simulink model "TVModel"  (R2022a)
settings: Solver=FixedStepDiscrete  StartTime=0.0  StopTime=10.0  FixedStep=0.02  MaxStep=0.01  RelTol=1e-3
undefined symbols (not defined in the file or in its folder): MB, TV, TV_OLD
libraries: simulink x22, simulink_extras x14, slpidlib x8, fuzblock x5, controlLib x4, dspstat3 x4, eeGeneralControl x3, cstblocks x3, eeSlidingModeController x1, sharedTrackingLibrary x1
(part 4 of 8)

== system TVModel/Subsystem/Subsystem1/Torque Distribution/Reference Tracking/YRD_LUT_-3 ==
  front_wheel_angle : Inport
  vx : Inport  Port=2
  Action Port : ActionPort  ActionPortLabel=elseif(u1 ==4)
  Abs : Abs  SaturateOnIntegerOverflow=off
  Cast3 : DataTypeConversion  Commented=on  OutDataTypeStr=single  SaturateOnIntegerOverflow=off  RndMeth=Floor
  Divide : Product  Inputs=*/
  Divide1 : Product  Inputs=*/
  Divide2 : Product  Inputs=**
  LUT_-3 : Lookup_n-D  BreakpointsForDimension1=TV.LUT.Yrd_LUT.LUT_vectors.delta_vector  BreakpointsForDimension2=TV.LUT.Yrd_LUT.LUT_vectors.v_vector  Table=single(TV.LUT.Yrd_LUT.LUT_neg3.ay_matrix)  InternalRulePriority=Speed  RndMeth=Simplest
      settings: InputPortMap=u0,u1
  Saturation : Saturate  UpperLimit=inf  LowerLimit=3
  yrd : Outport
  wires:
  front_wheel_angle/1 -> Divide1/1, Abs/1
  Abs/1 -> Divide1/2, LUT_-3/1  "absolute_front_wheel_angle"
  Divide/1 -> Divide2/2
  LUT_-3/1 -> Divide/1  "a"
  vx/1 -> Saturation/1
  Saturation/1 -> Divide/2, LUT_-3/2  "vx"
  Divide2/1 -> yrd/1  "yrd"
  Divide1/1 -> Divide2/1  "normalized_front_wheel_angle"

== system TVModel/Subsystem/Subsystem1/Torque Distribution/Reference Tracking/YRD_LUT_0 ==
  front_wheel_angle : Inport
  vx : Inport  Port=2
  Action Port : ActionPort  ActionPortLabel=elseif(u1 ==2)
  Abs : Abs  SaturateOnIntegerOverflow=off
  Cast : DataTypeConversion  Commented=on  OutDataTypeStr=single  SaturateOnIntegerOverflow=off  RndMeth=Floor
  Divide : Product  Inputs=*/
  Divide1 : Product  Inputs=*/
  Divide2 : Product  Inputs=**
  LUT_0 : Lookup_n-D  BreakpointsForDimension1=TV.LUT.Yrd_LUT.LUT_vectors.delta_vector  BreakpointsForDimension2=TV.LUT.Yrd_LUT.LUT_vectors.v_vector  Table=single(TV.LUT.Yrd_LUT.LUT_0.ay_matrix)  InternalRulePriority=Speed  RndMeth=Simplest
      settings: InputPortMap=u0,u1
  Saturation : Saturate  UpperLimit=inf  LowerLimit=3
  yrd : Outport
  wires:
  front_wheel_angle/1 -> Divide1/1, Abs/1
  Saturation/1 -> Divide/2, LUT_0/2  "vx"
  Abs/1 -> Divide1/2, LUT_0/1  "absolute_front_wheel_angle"
  Divide2/1 -> yrd/1  "yrd"
  vx/1 -> Saturation/1
  Divide/1 -> Divide2/2
  Divide1/1 -> Divide2/1  "normalized_front_wheel_angle"
  LUT_0/1 -> Divide/1

== system TVModel/Subsystem/Subsystem1/Torque Distribution/Reference Tracking/YRD_LUT_1 ==
  front_wheel_angle : Inport
  vx : Inport  Port=2
  Action Port : ActionPort  ActionPortLabel=if(u1 == 1)
  Abs : Abs  SaturateOnIntegerOverflow=off
  Cast3 : DataTypeConversion  Commented=on  OutDataTypeStr=single  SaturateOnIntegerOverflow=off  RndMeth=Floor
  Divide : Product  Inputs=*/
  Divide1 : Product  Inputs=*/
  Divide2 : Product  Inputs=**
  LUT_1 : Lookup_n-D  BreakpointsForDimension1=TV.LUT.Yrd_LUT.LUT_vectors.delta_vector  BreakpointsForDimension2=TV.LUT.Yrd_LUT.LUT_vectors.v_vector  Table=single(TV.LUT.Yrd_LUT.LUT_1.ay_matrix)  InternalRulePriority=Speed  RndMeth=Simplest
      settings: InputPortMap=u0,u1
  Saturation : Saturate  UpperLimit=inf  LowerLimit=3
  yrd : Outport
  wires:
  front_wheel_angle/1 -> Divide1/1, Abs/1
  LUT_1/1 -> Divide/1
  vx/1 -> Saturation/1
  Divide1/1 -> Divide2/1  "normalized_front_wheel_angle"
  Divide2/1 -> yrd/1  "yrd"
  Abs/1 -> Divide1/2, LUT_1/1  "absolute_front_wheel_angle"
  Saturation/1 -> Divide/2, LUT_1/2  "vx"
  Divide/1 -> Divide2/2

== system TVModel/Subsystem/Subsystem1/Torque Distribution/Reference Tracking/YRD_LUT_2 ==
  front_wheel_angle : Inport
  vx : Inport  Port=2
  Action Port : ActionPort  ActionPortLabel=elseif(u1 ==2)
  Abs : Abs  SaturateOnIntegerOverflow=off
  Cast : DataTypeConversion  Commented=on  OutDataTypeStr=single  SaturateOnIntegerOverflow=off  RndMeth=Floor
  Divide : Product  Inputs=*/
  Divide1 : Product  Inputs=*/
  Divide2 : Product  Inputs=**
  LUT_0 : Lookup_n-D  BreakpointsForDimension1=TV.LUT.Yrd_LUT.LUT_vectors.delta_vector  BreakpointsForDimension2=TV.LUT.Yrd_LUT.LUT_vectors.v_vector  Table=single(TV.LUT.Yrd_LUT.LUT_0.ay_matrix)  InternalRulePriority=Speed  RndMeth=Simplest
      settings: InputPortMap=u0,u1
  Saturation : Saturate  UpperLimit=inf  LowerLimit=3
  yrd : Outport
  wires:
  LUT_0/1 -> Divide/1
  Divide1/1 -> Divide2/1  "normalized_front_wheel_angle"
  Divide/1 -> Divide2/2
  vx/1 -> Saturation/1
  Divide2/1 -> yrd/1  "yrd"
  Abs/1 -> LUT_0/1, Divide1/2  "absolute_front_wheel_angle"
  Saturation/1 -> LUT_0/2, Divide/2  "vx"
  front_wheel_angle/1 -> Abs/1, Divide1/1

== system TVModel/Subsystem/Subsystem1/Torque Distribution/Reference Tracking/YRD_LUT_3 ==
  front_wheel_angle : Inport
  vx : Inport  Port=2
  Action Port : ActionPort  ActionPortLabel=if(u1 == 1)
  Abs : Abs  SaturateOnIntegerOverflow=off
  Cast3 : DataTypeConversion  Commented=on  OutDataTypeStr=single  SaturateOnIntegerOverflow=off  RndMeth=Floor
  Divide : Product  Inputs=*/
  Divide1 : Product  Inputs=*/
  Divide2 : Product  Inputs=**
  LUT_1 : Lookup_n-D  BreakpointsForDimension1=TV.LUT.Yrd_LUT.LUT_vectors.delta_vector  BreakpointsForDimension2=TV.LUT.Yrd_LUT.LUT_vectors.v_vector  Table=single(TV.LUT.Yrd_LUT.LUT_1.ay_matrix)  InternalRulePriority=Speed  RndMeth=Simplest
      settings: InputPortMap=u0,u1
  Saturation : Saturate  UpperLimit=inf  LowerLimit=3
  yrd : Outport
  wires:
  Divide/1 -> Divide2/2
  Saturation/1 -> LUT_1/2, Divide/2  "vx"
  Abs/1 -> LUT_1/1, Divide1/2  "absolute_front_wheel_angle"
  Divide2/1 -> yrd/1  "yrd"
  Divide1/1 -> Divide2/1  "normalized_front_wheel_angle"
  vx/1 -> Saturation/1
  LUT_1/1 -> Divide/1
  front_wheel_angle/1 -> Abs/1, Divide1/1

== system TVModel/Subsystem/Subsystem1/Torque Limits/Torque Limits Positive/Torque_Curve ==
  omega_wheels : Inport
  voltage [ID380] : Inport  Port=2
  torque_map : Inport  Port=3
  2-D Lookup Table : Lookup_n-D  BreakpointsForDimension1=TV.LV.TORQUE.T_lim_pos.breakpoints1  BreakpointsForDimension2=TV.LV.TORQUE.T_lim_pos.breakpoints2  Table=TV.LV.TORQUE.T_lim_pos.table_data  ExtrapMethod=Clip  InternalRulePriority=Speed  OutDataTypeStr=double  RndMeth=Simplest
      settings: InputPortMap=u0,u1
  Constant : Constant  Value=0
  Constant1 : Constant  Value=TV.LV.TORQUE.T_peak_motor
  Constant2 : Constant  Value=TV.LV.TORQUE.T_nominal_motor
  Gain : Gain  Gain=TV.LV.TORQUE.T_nominal_motor/1000
  Gain4 : Gain  Gain=TV.CAR.Tau*60/(2*pi)
  Low-Pass Filter (Discrete or Continuous) : eeGeneralControl/Low-Pass Filter (Discrete or Continuous)  K=1  T=1/4/pi  B=inf  A=-inf  init_option=Inherited from block input  x0=0  Ts=TV.MPC.T/TV.MPC.N
  Multiport Switch : MultiPortSwitch  DataPortOrder=Specify indices  DataPortIndices={TV.LV.TORQUE.T_peak_setting,TV.LV.TORQUE.T_nominal_setting}  DiagnosticForDefault=None  SaturateOnIntegerOverflow=off  InputSameDT=off
  Saturation Dynamic : simulink/Discontinuities/Saturation Dynamic  OutMin=[]  OutMax=[]  OutDataTypeStr=Inherit: Same as second input  OutDataType=fixdt(1, 16)  OutScaling=2^-10  DoSatur=off
  Saturation1 : Saturate  UpperLimit=+inf  LowerLimit=0
  max_torque_available : Outport
  wires:
  Low-Pass Filter (Discrete or Continuous)/1 -> Saturation Dynamic/2
  omega_wheels/1 -> Gain4/1
  Constant/1 -> Saturation Dynamic/3
  torque_map/1 -> Multiport Switch/1
  Constant1/1 -> Multiport Switch/2
  Constant2/1 -> Multiport Switch/3
  Multiport Switch/1 -> Saturation Dynamic/1  "torque map selected"
  Saturation1/1 -> 2-D Lookup Table/1
  voltage [ID380]/1 -> 2-D Lookup Table/2
  Gain/1 -> Low-Pass Filter (Discrete or Continuous)/1
  2-D Lookup Table/1 -> Gain/1
  Gain4/1 -> Saturation1/1  "RPM_Motors"
  Saturation Dynamic/1 -> max_torque_available/1

== system TVModel/Subsystem/Subsystem1/Torque Limits/Torque Limits Regen/Torque_Curve ==
  omega_wheels : Inport
  voltage [ID380] : Inport  Port=2
  torque_map : Inport  Port=3
  2-D Lookup Table : Lookup_n-D  BreakpointsForDimension1=TV.LV.TORQUE.T_lim_pos.breakpoints1  BreakpointsForDimension2=TV.LV.TORQUE.T_lim_pos.breakpoints2  Table=TV.LV.TORQUE.T_lim_pos.table_data  ExtrapMethod=Clip  InternalRulePriority=Speed  OutDataTypeStr=double  RndMeth=Simplest
      settings: InputPortMap=u0,u1
  Constant : Constant  Value=0
  Constant1 : Constant  Value=TV.LV.TORQUE.T_peak_motor
  Constant2 : Constant  Value=TV.LV.TORQUE.T_nominal_motor
  Gain : Gain  Gain=TV.LV.TORQUE.T_nominal_motor/1000
  Gain4 : Gain  Gain=TV.CAR.Tau*60/(2*pi)
  Low-Pass Filter (Discrete or Continuous) : eeGeneralControl/Low-Pass Filter (Discrete or Continuous)  K=1  T=1/4/pi  B=inf  A=-inf  init_option=Inherited from block input  x0=0  Ts=TV.MPC.T/TV.MPC.N
  Multiport Switch : MultiPortSwitch  DataPortOrder=Specify indices  DataPortIndices={TV.LV.TORQUE.T_peak_setting,TV.LV.TORQUE.T_nominal_setting}  DiagnosticForDefault=None  SaturateOnIntegerOverflow=off  InputSameDT=off
  Saturation Dynamic : simulink/Discontinuities/Saturation Dynamic  OutMin=[]  OutMax=[]  OutDataTypeStr=Inherit: Same as second input  OutDataType=fixdt(1, 16)  OutScaling=2^-10  DoSatur=off
  Saturation1 : Saturate  UpperLimit=+inf  LowerLimit=0
  max_torque_available : Outport
  wires:
  Low-Pass Filter (Discrete or Continuous)/1 -> Saturation Dynamic/2
  omega_wheels/1 -> Gain4/1
  Constant/1 -> Saturation Dynamic/3
  torque_map/1 -> Multiport Switch/1
  Constant1/1 -> Multiport Switch/2
  Constant2/1 -> Multiport Switch/3
  Multiport Switch/1 -> Saturation Dynamic/1  "torque map selected"
  Saturation1/1 -> 2-D Lookup Table/1
  voltage [ID380]/1 -> 2-D Lookup Table/2
  Gain/1 -> Low-Pass Filter (Discrete or Continuous)/1
  2-D Lookup Table/1 -> Gain/1
  Gain4/1 -> Saturation1/1  "RPM_Motors"
  Saturation Dynamic/1 -> max_torque_available/1

== system TVModel/Subsystem/Subsystem1/Torque Limits/Torque Request/T_Req_Acceleration ==
  throttle : Inport
  torque_map : Inport  Port=2
  Constant : Constant  Value=0
  Constant1 : Constant
  Constant2 : Constant  Value=0
  Data Store General_Params : DataStoreRead  DataStoreName=General_Params  DataStoreElements=General_Params.ThrottleThresh  IndexOptions=Index vector (dialog)  Indices=1  OutputSizes=1
  Data Store General_Params1 : DataStoreRead  DataStoreName=General_Params  DataStoreElements=General_Params.ThrottleThresh  IndexOptions=Index vector (dialog)  Indices=1  OutputSizes=1
  Less Than : RelationalOperator  Operator=>  OutDataTypeStr=boolean  RndMeth=Simplest  InputSameDT=off
  Map_Selector : MultiPortSwitch  DataPortOrder=Specify indices  DataPortIndices={TV.LV.TORQUE.T_peak_setting,TV.LV.TORQUE.T_nominal_setting}  DiagnosticForDefault=None  SaturateOnIntegerOverflow=off  InputSameDT=off
  Mux : Mux  Inputs=3
  Switch : Switch  Criteria=u2 > Threshold  SaturateOnIntegerOverflow=off  InputSameDT=off
  T_nominal_wheel_LUT : Lookup_n-D  NumberOfTableDimensions=1  BreakpointsForDimension1Source=Input port  BreakpointsForDimension1=[-5:5]  Table=[0,0, 4*TV.LV.TORQUE.T_nominal_wheel]  InternalRulePriority=Speed  RndMeth=Simplest
      settings: InputPortMap=u0,p5
  T_peak_wheel_LUT : Lookup_n-D  NumberOfTableDimensions=1  BreakpointsForDimension1Source=Input port  BreakpointsForDimension1=[-5:5]  Table=[0,0, 4*TV.LV.TORQUE.T_peak_wheel]  InternalRulePriority=Speed  RndMeth=Simplest
      settings: InputPortMap=u0,p5
  "t_req " : Outport
  wires:
  throttle/1 -> T_nominal_wheel_LUT/1, Less Than/1, T_peak_wheel_LUT/1  "throttle"
  Map_Selector/1 -> Switch/1  "t"
  Data Store General_Params1/1 -> Less Than/2  "throttle_thresh"
  Less Than/1 -> Switch/2  "throttle"
  Switch/1 -> "t_req "/1
  Constant/1 -> Switch/3
  T_nominal_wheel_LUT/1 -> Map_Selector/3
  T_peak_wheel_LUT/1 -> Map_Selector/2
  torque_map/1 -> Map_Selector/1  "torque_map"
  Mux/1 -> T_nominal_wheel_LUT/2, T_peak_wheel_LUT/2
  Data Store General_Params/1 -> Mux/2  "throttle_thresh"
  Constant1/1 -> Mux/3
  Constant2/1 -> Mux/1

== system TVModel/Subsystem/Subsystem1/Torque Limits/Torque Request/T_Req_Braking ==
  brake : Inport
  1-D Lookup Table : Lookup_n-D  NumberOfTableDimensions=1  BreakpointsForDimension1Source=Input port  BreakpointsForDimension1=[-5:5]  Table=[0,1]  InternalRulePriority=Speed  RndMeth=Simplest
      settings: InputPortMap=u0,p5
  Constant : Constant
  Data Store Read : DataStoreRead  DataStoreName=General_Params  DataStoreElements=General_Params.BrakeThresh  IndexOptions=Index vector (dialog)  Indices=1  OutputSizes=1
  Gain_Max_Torque_Needed : Gain  Gain=-4*TV.LV.TORQUE.T_nominal_wheel
  Mux : Mux  Inputs=2
  Saturation_Brake : Saturate  UpperLimit=1  LowerLimit=0
  "t_req " : Outport
  wires:
  Gain_Max_Torque_Needed/1 -> "t_req "/1  "t_req"
  brake/1 -> 1-D Lookup Table/1  "brake"
  1-D Lookup Table/1 -> Saturation_Brake/1  "brake"
  Saturation_Brake/1 -> Gain_Max_Torque_Needed/1  "brake"
  Data Store Read/1 -> Mux/1
  Constant/1 -> Mux/2
  Mux/1 -> 1-D Lookup Table/2

== system TVModel/Subsystem/Subsystem1/Slip Control/Traction Control/Load Transfer calculation/Fz FL ==
  In Bus Element : Inport  PortName=dynamics_data  Element=ay
  In Bus Element1 : Inport  PortName=dynamics_data  Element=vx
  In Bus Element2 : Inport  PortName=dynamics_data  Element=ax
  Drag moment : Gain  Gain=0.5*TV.CAR.rho*TV.CAR.CdA*TV.CAR.hcop/TV.CAR.wb*0.5
  Lateral Load Transfer : Gain  Gain=TV.CAR.m/TV.CAR.tf*TV.CAR.hcog*0.5*0.5
  Lift Force : Gain  Gain=0.5*TV.CAR.rho*TV.CAR.ClA*(1-TV.CAR.xcop/TV.CAR.wb)*0.5
  Longitudinal Load Transfer : Gain  Gain=TV.CAR.m/TV.CAR.wb*TV.CAR.hcog*0.5
  Square1 : Math  Operator=square
  Square2 : Math  Operator=square
  Static Load Front : Constant  Value=TV.CAR.Fzf
  Subtract : Sum  Inputs=+++-+
  Unary Minus : UnaryMinus
  Unary Minus1 : UnaryMinus
  TV_Info : Outport
  wires:
  Unary Minus1/1 -> Longitudinal Load Transfer/1
  Unary Minus/1 -> Lateral Load Transfer/1
  In Bus Element/1 -> Unary Minus/1
  Subtract/1 -> TV_Info/1
  Drag moment/1 -> Subtract/4
  Static Load Front/1 -> Subtract/1
  Square1/1 -> Lift Force/1
  Lateral Load Transfer/1 -> Subtract/2
  Longitudinal Load Transfer/1 -> Subtract/5
  In Bus Element2/1 -> Unary Minus1/1
  Square2/1 -> Drag moment/1
  In Bus Element1/1 -> Square2/1, Square1/1
  Lift Force/1 -> Subtract/3

== system TVModel/Subsystem/Subsystem1/Slip Control/Traction Control/Load Transfer calculation/Fz FR ==
  In Bus Element : Inport  PortName=dynamics_data  Element=ay
  In Bus Element1 : Inport  PortName=dynamics_data  Element=vx
  In Bus Element2 : Inport  PortName=dynamics_data  Element=ax
  Drag moment : Gain  Gain=0.5*TV.CAR.rho*TV.CAR.CdA*TV.CAR.hcop/TV.CAR.wb*0.5
  Lateral Load Transfer : Gain  Gain=TV.CAR.m/TV.CAR.tf*TV.CAR.hcog*0.5*0.5
  Lift Force : Gain  Gain=0.5*TV.CAR.rho*TV.CAR.ClA*(1 - TV.CAR.xcop/TV.CAR.wb)*0.5
  Longitudinal Load Transfer : Gain  Gain=TV.CAR.m/TV.CAR.wb*TV.CAR.hcog*0.5
  Square1 : Math  Operator=square
  Square2 : Math  Operator=square
  Static Load Front : Constant  Value=TV.CAR.Fzf
  Subtract : Sum  Inputs=+-+-+
  Unary Minus : UnaryMinus
  Unary Minus1 : UnaryMinus
  TV_Info : Outport
  wires:
  Unary Minus1/1 -> Longitudinal Load Transfer/1
  Unary Minus/1 -> Lateral Load Transfer/1
  Subtract/1 -> TV_Info/1
  Drag moment/1 -> Subtract/4
  In Bus Element/1 -> Unary Minus/1
  In Bus Element1/1 -> Square1/1, Square2/1
  Static Load Front/1 -> Subtract/1
  Square1/1 -> Lift Force/1
  Lateral Load Transfer/1 -> Subtract/2
  Longitudinal Load Transfer/1 -> Subtract/5
  In Bus Element2/1 -> Unary Minus1/1
  Lift Force/1 -> Subtract/3
  Square2/1 -> Drag moment/1

== system TVModel/Subsystem/Subsystem1/Slip Control/Traction Control/Load Transfer calculation/Fz RL ==
  In Bus Element : Inport  PortName=dynamics_data  Element=ay
  In Bus Element1 : Inport  PortName=dynamics_data  Element=vx
  In Bus Element2 : Inport  PortName=dynamics_data  Element=ax
  Drag moment : Gain  Gain=0.5*TV.CAR.rho*TV.CAR.CdA*TV.CAR.hcop/TV.CAR.wb*0.5
  Lateral Load Transfer : Gain  Gain=TV.CAR.m/TV.CAR.tr*TV.CAR.hcog*0.5*0.5
  Lift Force : Gain  Gain=0.5*TV.CAR.rho*TV.CAR.ClA*(TV.CAR.xcop/TV.CAR.wb)*0.5
  Longitudinal Load Transfer : Gain  Gain=TV.CAR.m/TV.CAR.wb*TV.CAR.hcog*0.5
  Square1 : Math  Operator=square
  Square2 : Math  Operator=square
  Static Load Front : Constant  Value=TV.CAR.Fzr
  Subtract : Sum  Inputs=++++-
  Unary Minus : UnaryMinus
  Unary Minus1 : UnaryMinus
  TV_Info : Outport
  wires:
  Unary Minus1/1 -> Longitudinal Load Transfer/1
  Unary Minus/1 -> Lateral Load Transfer/1
  Subtract/1 -> TV_Info/1
  Drag moment/1 -> Subtract/4
  In Bus Element/1 -> Unary Minus/1
  Static Load Front/1 -> Subtract/1
  Square1/1 -> Lift Force/1
  Lateral Load Transfer/1 -> Subtract/2
  Longitudinal Load Transfer/1 -> Subtract/5
  In Bus Element2/1 -> Unary Minus1/1
  Lift Force/1 -> Subtract/3
  Square2/1 -> Drag moment/1
  In Bus Element1/1 -> Square2/1, Square1/1

== system TVModel/Subsystem/Subsystem1/Slip Control/Traction Control/Load Transfer calculation/Fz RR ==
  In Bus Element : Inport  PortName=dynamics_data  Element=ay
  In Bus Element1 : Inport  PortName=dynamics_data  Element=vx
  In Bus Element2 : Inport  PortName=dynamics_data  Element=ax
  Drag moment : Gain  Gain=0.5*TV.CAR.rho*TV.CAR.CdA*TV.CAR.hcop/TV.CAR.wb*0.5
  Lateral Load Transfer : Gain  Gain=TV.CAR.m/TV.CAR.tr*TV.CAR.hcog*0.5*0.5
  Lift Force : Gain  Gain=0.5*TV.CAR.rho*TV.CAR.ClA*(TV.CAR.xcop/TV.CAR.wb)*0.5
  Longitudinal Load Transfer : Gain  Gain=TV.CAR.m/TV.CAR.wb*TV.CAR.hcog*0.5
  Square1 : Math  Operator=square
  Square2 : Math  Operator=square
  Static Load Front : Constant  Value=TV.CAR.Fzr
  Subtract : Sum  Inputs=+-++-
  Unary Minus : UnaryMinus
  Unary Minus1 : UnaryMinus
  TV_Info : Outport
  wires:
  Unary Minus1/1 -> Longitudinal Load Transfer/1
  Unary Minus/1 -> Lateral Load Transfer/1
  Subtract/1 -> TV_Info/1
  Drag moment/1 -> Subtract/4
  In Bus Element/1 -> Unary Minus/1
  In Bus Element1/1 -> Square1/1, Square2/1
  Static Load Front/1 -> Subtract/1
  Square1/1 -> Lift Force/1
  Lateral Load Transfer/1 -> Subtract/2
  Longitudinal Load Transfer/1 -> Subtract/5
  In Bus Element2/1 -> Unary Minus1/1
  Lift Force/1 -> Subtract/3
  Square2/1 -> Drag moment/1

== system TVModel/Subsystem/Subsystem1/Slip Control/Traction Control/S-R Flip Flops/Subsystem ==
  In1 : Inport
  In2 : Inport  Port=2
  Demux : Demux
  Demux1 : Demux
  Mux : Mux
  S-R Flip-Flop{,1..3} (4 alike) : simulink_extras/Flip Flops/S-R Flip-Flop  initial_condition=0
  Out1 : Outport
  wires:
  Demux1/1 -> S-R Flip-Flop/2
  Demux1/2 -> S-R Flip-Flop1/2
  Demux/4 -> S-R Flip-Flop3/1
  Demux/1 -> S-R Flip-Flop/1
  In1/1 -> Demux/1
  Demux1/3 -> S-R Flip-Flop2/2
  Demux/2 -> S-R Flip-Flop1/1
  Demux1/4 -> S-R Flip-Flop3/2
  S-R Flip-Flop2/1 -> Mux/3
  Demux/3 -> S-R Flip-Flop2/1
  S-R Flip-Flop3/1 -> Mux/4
  In2/1 -> Demux1/1
  Mux/1 -> Out1/1
  S-R Flip-Flop1/1 -> Mux/2
  S-R Flip-Flop/1 -> Mux/1

== system TVModel/Subsystem/Subsystem1/Slip Control/Traction Control/Slip Control/ABS ==
  eps_target : Inport
  eps : Inport  Port=2
  Reset Signal : Inport  Port=3
  T_actual : Inport  Port=4  PortDimensions=4
  T_limit : Inport  Port=5
  RTD_flag : Inport  Port=6
  Activation logic : Stateflow chart  TreatAsAtomicUnit=on
  Constant : Constant  Value=0.01
  Constant1 : Constant  Value=57
  Constant2 : Constant  Value=2845
  Constant3 : Constant  Value=4.9
  Constant4 : Constant  Value=-21
  Constant5 : Constant  Value=0.9
  Gain : Gain  Gain=-1
  Minus : Sum  Inputs=+-
  PID Controller5 : slpidlib/PID Controller  Controller=PI  Form=Parallel  TimeDomain=Discrete-time  UseExternalTs=off  SampleTime=0.02  IntegratorMethod=Forward Euler  FilterMethod=Forward Euler  ControllerParametersSource=external  P=57  I=2845  UseKiTs=off  D=0  N=63.8249907657072  UseFilter=off  TunerSelectOption=Transfer Function Based (PID Tuner App)  InitialConditionSource=internal  InitialConditionForIntegrator=0  InitialConditionForFilter=0  DifferentiatorICPrevScaledInput=0  ExternalReset=rising  TrackingMode=on  Kt=TV_OLD.LV.GEN.slipKt  LimitOutput=on  SatLimitsSource=external  UpperSaturationLimit=0  LowerSaturationLimit=-TV_OLD.LV.Tpeak  LinearizeAsGain=on  AntiWindupMode=clamping  Kb=1  POutMin=[]  POutMax=[]  IOutMin=[]  IOutMax=[]  DOutMin=[]  DOutMax=[]  NOutMin=[]  NOutMax=[]  SumOutMin=[]  SumOutMax=[]  SaturationOutMin=[]  SaturationOutMax=[]  PParamMin=[]  PParamMax=[]  IParamMin=[]  IParamMax=[]  DParamMin=[]  DParamMax=[]  NParamMin=[]  NParamMax=[]  KbParamMin=[]  KbParamMax=[]  KtParamMin=[]  KtParamMax=[]  KbOutMin=[]  KbOutMax=[]  KtOutMin=[]  KtOutMax=[]  IntegratorOutMin=[]  IntegratorOutMax=[]  FilterOutMin=[]  FilterOutMax=[]  SumI1OutMin=[]  SumI1OutMax=[]  SumI2OutMin=[]  SumI2OutMax=[]  SumI3OutMin=[]  SumI3OutMax=[]  SumI4OutMin=[]  SumI4OutMax=[]  SumDOutMin=[]  SumDOutMax=[]  DifferentiatorOutMin=[]  DifferentiatorOutMax=[]  FilterDiffOutCoefMin=[]  FilterDiffOutCoefMax=[]  ReciprocalOutMin=[]  ReciprocalOutMax=[]  SumDenOutMin=[]  SumDenOutMax=[]  SumNumOutMin=[]  SumNumOutMax=[]  DivideOutMin=[]  DivideOutMax=[]  UdiffTsProdOutMin=[]  UdiffTsProdOutMax=[]  NTsProdOutMin=[]  NTsProdOutMax=[]  UintegralTsProdOutMin=[]  UintegralTsProdOutMax=[]  UngainTsProdOutMin=[]  UngainTsProdOutMax=[]  IntegratorContinuousStateAttributes=''  IntegratorStateMustResolveToSignalObject=off  IntegratorRTWStateStorageClass=Auto  FilterContinuousStateAttributes=''  FilterStateMustResolveToSignalObject=off  FilterRTWStateStorageClass=Auto  ParallelPVariant=ExternalParameters  IdealPVariant=Disabled  IVariant=ExternalParameters  DVariant=Disabled  IntegratorVariant=Discrete  SatVariant=External  AWVariant=DiscClampingParallel  PCopyVariant=Disabled  TRVariant=Enabled  FdbkBlocksVariant=Forward  IdealPFdbkVariant=Disabled  SatFdbkVariant=Disabled  DerivativeFilterVariant=Disabled  NVariant=Disabled  NCopyVariant=Disabled_SignalSpec  FilterICVariant=Disabled  IntegratorICVariant=InternalICs  ExternalResetVariant=ExternalReset  TRSumVariant=TrackingMode  SumFdbkVariant=Disabled  SumVariant=Sum_PI  TsampFilterVariant=InternalTs  TsampNgainVariant=Passthrough  TsampIntegralVariant=Passthrough  ExternalSaturationOutDataTypeStr=Inherit: Same as second input  aMode=0
  Unit Delay : UnitDelay  InitialCondition=zeros(4,1)  SampleTime=-1  HasFrameUpgradeWarning=on
  Tmin : Outport
  wires:
  Constant2/1 -> PID Controller5/3
  Constant1/1 -> PID Controller5/2
  [ResetSignal] -> Activation logic/6(TC_flag)
  [ResetSignal] -> PID Controller5/4
  Reset Signal/1 -> [ResetSignal]
  [eps] -> Activation logic/3(eps)
  [eps] -> Minus/2
  eps/1 -> [eps]
  [eps_target] -> Activation logic/2(epsTarget)
  eps_target/1 -> [eps_target]
  Minus/1 -> PID Controller5/1
  Activation logic/1(T_min) -> Tmin/1, Unit Delay/1, PID Controller5/7
  T_actual/1 -> Activation logic/4(T_actual)
  Unit Delay/1 -> Activation logic/7(Tmin_old)
  [eps_target] -> Minus/1
  PID Controller5/1 -> Activation logic/1(Tmin_PI)  "Tmin_PI"
  T_limit/1 -> Activation logic/5(T_limit)
  Constant/1 -> Activation logic/8(slipNoise)
  Constant3/1 -> Gain/1
  Gain/1 -> PID Controller5/5
  Constant4/1 -> PID Controller5/6
  Constant5/1 -> Activation logic/9(slipDeactPerc)
  RTD_flag/1 -> Activation logic/10(RTD_flag)

== system TVModel/Subsystem/Subsystem1/Slip Control/Traction Control/Slip Control/Reset ABS ==
  V : Inport
  throttle : Inport  Port=2
  brake : Inport  Port=3
  TC_setting : Inport  Port=4
  RTD : Inport  Port=5
  AND : Logic  Inputs=3  IconShape=distinctive  AllPortsSameDT=off  OutDataTypeStr=boolean
  Constant : Constant  Value=0
  Constant1 : Constant  Value=0
  Constant2 : Constant  Value=3
  Data Store Read1 : DataStoreRead  Commented=on  DataStoreName=thresholds  DataStoreElements=thresholds.THROTTLE_RELAY_AMP#thresholds.THROTTLE_NOISE#thresholds.BRAKE_RELAY_AMP#thresholds.BRAKE_NOISE  IndexOptions=Index vector (dialog)  Indices=1  OutputSizes=1
  NOT : Logic  Commented=on  Operator=NOT  IconShape=distinctive  AllPortsSameDT=off  OutDataTypeStr=boolean
  Relational Operator : RelationalOperator  Operator=>  OutDataTypeStr=boolean  RndMeth=Simplest  InputSameDT=off
  Relational Operator3 : RelationalOperator  Operator=>  OutDataTypeStr=boolean  RndMeth=Simplest  InputSameDT=off
  Relational Operator4 : RelationalOperator  Operator=>  OutDataTypeStr=boolean  RndMeth=Simplest  InputSameDT=off
  Variable Amplitude Relay : controlLib/Variable Amplitude Relay  Commented=on  SystemSampleTime=-1  VariantActivationTime=update diagram  Latency=0  AutoFrameSizeCalculation=off
      settings: SourceProductName=VCU Library
  Variable Amplitude Relay1 : controlLib/Variable Amplitude Relay  Commented=on  SystemSampleTime=-1  VariantActivationTime=update diagram  Latency=0  AutoFrameSizeCalculation=off
      settings: SourceProductName=VCU Library
  resetSignal : Outport
  wires:
  Variable Amplitude Relay/1 -> NOT/1
  brake/1 -> Variable Amplitude Relay/3
  throttle/1 -> Variable Amplitude Relay1/3
  Data Store Read1/2 -> Variable Amplitude Relay1/2
  Data Store Read1/3 -> Variable Amplitude Relay/1
  Data Store Read1/4 -> Variable Amplitude Relay/2
  AND/1 -> resetSignal/1
  Relational Operator4/1 -> AND/3
  Relational Operator3/1 -> AND/2
  Relational Operator/1 -> AND/1
  RTD/1 -> Relational Operator4/1
  Constant1/1 -> Relational Operator4/2
  Constant/1 -> Relational Operator3/2
  TC_setting/1 -> Relational Operator3/1
  Data Store Read1/1 -> Variable Amplitude Relay1/1
  V/1 -> Relational Operator/1
  Constant2/1 -> Relational Operator/2

== system TVModel/Subsystem/Subsystem1/Slip Control/Traction Control/Slip Control/Reset TC ==
  V : Inport
  throttle : Inport  Port=2
  brake : Inport  Port=3
  TC_setting : Inport  Port=4
  RTD : Inport  Port=5
  AND : Logic  Inputs=5  IconShape=distinctive  AllPortsSameDT=off  OutDataTypeStr=boolean
  Constant : Constant  Value=0
  Constant1 : Constant  Value=0
  Constant2 : Constant  Value=3
  Constant3 : Constant  Value=0.01
  Constant4 : Constant  Value=0.05
  Constant5 : Constant  Value=0.01
  Constant6 : Constant  Value=0.1
  NOT : Logic  Operator=NOT  IconShape=distinctive  AllPortsSameDT=off  OutDataTypeStr=boolean
  Relational Operator : RelationalOperator  Operator=>  OutDataTypeStr=boolean  RndMeth=Simplest  InputSameDT=off
  Relational Operator3 : RelationalOperator  Operator=>  OutDataTypeStr=boolean  RndMeth=Simplest  InputSameDT=off
  Relational Operator4 : RelationalOperator  Operator=>  OutDataTypeStr=boolean  RndMeth=Simplest  InputSameDT=off
  Variable Amplitude Relay : controlLib/Variable Amplitude Relay  SystemSampleTime=-1  VariantActivationTime=update diagram  Latency=0  AutoFrameSizeCalculation=off
      settings: SourceProductName=VCU Library
  Variable Amplitude Relay1 : controlLib/Variable Amplitude Relay  SystemSampleTime=-1  VariantActivationTime=update diagram  Latency=0  AutoFrameSizeCalculation=off
      settings: SourceProductName=VCU Library
  resetSignal : Outport
  wires:
  Constant2/1 -> Relational Operator/2
  V/1 -> Relational Operator/1
  Constant3/1 -> Variable Amplitude Relay1/1
  TC_setting/1 -> Relational Operator3/1
  Constant/1 -> Relational Operator3/2
  Constant1/1 -> Relational Operator4/2
  RTD/1 -> Relational Operator4/1
  Relational Operator/1 -> AND/1
  Variable Amplitude Relay1/1 -> AND/2
  NOT/1 -> AND/3
  Relational Operator3/1 -> AND/4
  Relational Operator4/1 -> AND/5
  AND/1 -> resetSignal/1
  Constant6/1 -> Variable Amplitude Relay/2
  Constant5/1 -> Variable Amplitude Relay/1
  Constant4/1 -> Variable Amplitude Relay1/2
  throttle/1 -> Variable Amplitude Relay1/3
  brake/1 -> Variable Amplitude Relay/3
  Variable Amplitude Relay/1 -> NOT/1

== system TVModel/Subsystem/Subsystem1/Slip Control/Traction Control/Slip Control/Slip computation ==
  <Vx> : Inport
  <Vy> : Inport  Port=2
  <Yaw Rate> : Inport  Port=3
  <deltaL> : Inport  Port=4
  <deltaR> : Inport  Port=5
  Constant : Constant  Value=3
  Constant1 : Constant  Value=1.53/2
  Constant2 : Constant  Value=1.27
  MATLAB Function2 : MATLAB Function  TreatAsAtomicUnit=on
  Vx_FL : Outport
  Vx_FR : Outport  Port=2
  Vx_RL : Outport  Port=3
  Vx_RR : Outport  Port=4
  alpha_FL : Outport  Port=5
  alpha_FR : Outport  Port=6
  alpha_RL : Outport  Port=7
  alpha_RR : Outport  Port=8
  wires:
  <deltaR>/1 -> MATLAB Function2/5(delta_R)
  <deltaL>/1 -> MATLAB Function2/4(delta_L)
  MATLAB Function2/8(alpha_RR) -> alpha_RR/1
  Constant1/1 -> MATLAB Function2/7(b), MATLAB Function2/6(a)
  MATLAB Function2/2(V_FR) -> Vx_FR/1
  MATLAB Function2/1(V_FL) -> Vx_FL/1
  <Vy>/1 -> MATLAB Function2/2(Vy)
  MATLAB Function2/3(V_RL) -> Vx_RL/1
  MATLAB Function2/4(V_RR) -> Vx_RR/1
  MATLAB Function2/5(alpha_FL) -> alpha_FL/1
  <Yaw Rate>/1 -> MATLAB Function2/3(phi_dot)
  MATLAB Function2/7(alpha_RL) -> alpha_RL/1
  <Vx>/1 -> MATLAB Function2/1(Vx)
  Constant2/1 -> MATLAB Function2/8(t)
  MATLAB Function2/6(alpha_FR) -> alpha_FR/1
  Constant/1 -> MATLAB Function2/9(Vx_min)

== system TVModel/Subsystem/Subsystem1/Slip Control/Traction Control/Slip Control/TC ==
  eps_target : Inport
  eps : Inport  Port=2
  Reset Signal : Inport  Port=3
  T_actual : Inport  Port=4  PortDimensions=4
  T_limit : Inport  Port=5
  RTD_flag : Inport  Port=6
  Activation logic : Stateflow chart  TreatAsAtomicUnit=on
  Constant1 : Constant  Value=57
  Constant2 : Constant  Value=2845
  Constant3 : Constant  Value=4.9
  Constant4 : Constant  Value=0.01
  Constant5 : Constant  Value=0.9
  Constant6 : Constant  Value=21
  Minus : Sum  Inputs=+-
  PID Controller5 : slpidlib/PID Controller  Controller=PI  Form=Parallel  TimeDomain=Discrete-time  UseExternalTs=off  SampleTime=0.02  IntegratorMethod=Forward Euler  FilterMethod=Forward Euler  ControllerParametersSource=external  P=57  I=2845  UseKiTs=off  D=0  N=63.8249907657072  UseFilter=off  TunerSelectOption=Transfer Function Based (PID Tuner App)  InitialConditionSource=internal  InitialConditionForIntegrator=0  InitialConditionForFilter=0  DifferentiatorICPrevScaledInput=0  ExternalReset=rising  TrackingMode=on  Kt=TV_OLD.LV.GEN.slipKt  LimitOutput=on  SatLimitsSource=external  UpperSaturationLimit=21*TV_OLD.CAR.tau  LowerSaturationLimit=5*TV_OLD.CAR.tau  LinearizeAsGain=on  AntiWindupMode=clamping  Kb=1  POutMin=[]  POutMax=[]  IOutMin=[]  IOutMax=[]  DOutMin=[]  DOutMax=[]  NOutMin=[]  NOutMax=[]  SumOutMin=[]  SumOutMax=[]  SaturationOutMin=[]  SaturationOutMax=[]  PParamMin=[]  PParamMax=[]  IParamMin=[]  IParamMax=[]  DParamMin=[]  DParamMax=[]  NParamMin=[]  NParamMax=[]  KbParamMin=[]  KbParamMax=[]  KtParamMin=[]  KtParamMax=[]  KbOutMin=[]  KbOutMax=[]  KtOutMin=[]  KtOutMax=[]  IntegratorOutMin=[]  IntegratorOutMax=[]  FilterOutMin=[]  FilterOutMax=[]  SumI1OutMin=[]  SumI1OutMax=[]  SumI2OutMin=[]  SumI2OutMax=[]  SumI3OutMin=[]  SumI3OutMax=[]  SumI4OutMin=[]  SumI4OutMax=[]  SumDOutMin=[]  SumDOutMax=[]  DifferentiatorOutMin=[]  DifferentiatorOutMax=[]  FilterDiffOutCoefMin=[]  FilterDiffOutCoefMax=[]  ReciprocalOutMin=[]  ReciprocalOutMax=[]  SumDenOutMin=[]  SumDenOutMax=[]  SumNumOutMin=[]  SumNumOutMax=[]  DivideOutMin=[]  DivideOutMax=[]  UdiffTsProdOutMin=[]  UdiffTsProdOutMax=[]  NTsProdOutMin=[]  NTsProdOutMax=[]  UintegralTsProdOutMin=[]  UintegralTsProdOutMax=[]  UngainTsProdOutMin=[]  UngainTsProdOutMax=[]  IntegratorContinuousStateAttributes=''  IntegratorStateMustResolveToSignalObject=off  IntegratorRTWStateStorageClass=Auto  FilterContinuousStateAttributes=''  FilterStateMustResolveToSignalObject=off  FilterRTWStateStorageClass=Auto  ParallelPVariant=ExternalParameters  IdealPVariant=Disabled  IVariant=ExternalParameters  DVariant=Disabled  IntegratorVariant=Discrete  SatVariant=External  AWVariant=DiscClampingParallel  PCopyVariant=Disabled  TRVariant=Enabled  FdbkBlocksVariant=Forward  IdealPFdbkVariant=Disabled  SatFdbkVariant=Disabled  DerivativeFilterVariant=Disabled  NVariant=Disabled  NCopyVariant=Disabled_SignalSpec  FilterICVariant=Disabled  IntegratorICVariant=InternalICs  ExternalResetVariant=ExternalReset  TRSumVariant=TrackingMode  SumFdbkVariant=Disabled  SumVariant=Sum_PI  TsampFilterVariant=InternalTs  TsampNgainVariant=Passthrough  TsampIntegralVariant=Passthrough  ExternalSaturationOutDataTypeStr=Inherit: Same as second input  aMode=0
  Unit Delay : UnitDelay  InitialCondition=zeros(4,1)  SampleTime=-1  HasFrameUpgradeWarning=on
  Tmax : Outport
  TC_Active : Outport  Port=2
  wires:
  Constant6/1 -> PID Controller5/5
  Constant3/1 -> PID Controller5/6
  Constant2/1 -> PID Controller5/3
  Constant1/1 -> PID Controller5/2
  [ResetSignal] -> Activation logic/6(TC_flag)
  [ResetSignal] -> PID Controller5/4
  [eps] -> Activation logic/3(eps)
  [eps_target] -> Activation logic/2(epsTarget)
  [eps_target] -> Minus/1
  Reset Signal/1 -> [ResetSignal]
  eps/1 -> [eps]
  eps_target/1 -> [eps_target]
  T_limit/1 -> Activation logic/5(T_limit)
  PID Controller5/1 -> Activation logic/1(Tmax_PI)  "Tmax_PI"
  Unit Delay/1 -> Activation logic/7(Tmax_old)
  [eps] -> Minus/2
  T_actual/1 -> Activation logic/4(T_actual)
  Activation logic/1(T_max) -> Unit Delay/1, PID Controller5/7, Tmax/1
  Minus/1 -> PID Controller5/1
  Constant4/1 -> Activation logic/8(slipNoise)
  Constant5/1 -> Activation logic/9(slipDeactPerc)
  RTD_flag/1 -> Activation logic/10(RTD_flag)
  Activation logic/2(TC_Active) -> TC_Active/1

== system TVModel/Subsystem/Subsystem1/Slip Control/Traction Control/Slip Control/epsTarget computation ==
  alpha wheels : Inport
  Constant : Constant  Value=0.96
  Constant1 : Constant
  Constant2 : Constant  Value=0.1*ones(4,1)
  Constant4 : Constant
  Minus : Sum  Inputs=+-
  Plus1 : Sum
  Product2 : Product
  Product3 : Product
  Terminator : Terminator
  epsTarget : Outport
  wires:
  Plus1/1 -> epsTarget/1  "epsTarget"
  alpha wheels/1 -> Terminator/1
  Minus/1 -> Product3/2
  Constant/1 -> Product2/1, Minus/2
  Constant1/1 -> Product3/1
  Constant4/1 -> Minus/1
  Constant2/1 -> Product2/2  "kappaTarget"
  Product2/1 -> Plus1/2
  Product3/1 -> Plus1/1

== system TVModel/Subsystem/Subsystem1/Slip Control/Traction Control/Slip Control/slip ratio ==
  v_wheels : Inport
  w : Inport  Port=2
  Constant : Constant  Value=3
  Discrete Derivative : simulink/Discrete/Discrete Derivative  gainval=1.0  ICPrevScaledInput=0.0  OutMin=[]  OutMax=[]  OutDataType=fixdt(1, 16)  OutScaling=2^-10  DoSatur=off
  Gain : Gain  Gain=0.235
  Gain2 : Gain  Gain=1/9.81
  MATLAB Function : MATLAB Function  TreatAsAtomicUnit=on
  kappa : Outport
  eta : Outport  Port=2
  wires:
  w/1 -> Gain/1
  Gain/1 -> Discrete Derivative/1, MATLAB Function/2(wR)  "ome_wheels"
  Discrete Derivative/1 -> Gain2/1
  Gain2/1 -> eta/1
  v_wheels/1 -> MATLAB Function/1(vx_wheels)  "v_wheels"
  MATLAB Function/1(k) -> kappa/1  "k_prova"
  Constant/1 -> MATLAB Function/3(vx_min)

== system TVModel/Subsystem/Subsystem1/Slip Control/Traction Control/Subsystem/Load Transfer Calculation ==
  In Bus Element : Inport  PortName=dynamics_data
  Fz FL : Subsystem
  Fz FR : Subsystem
  Fz RL : Subsystem
  Fz RR : Subsystem
  Mux : Mux
  Fz [4x1] : Outport
  wires:
  In Bus Element/1 -> Fz FL/1(dynamics_data), Fz FR/1(dynamics_data), Fz RL/1(dynamics_data), Fz RR/1(dynamics_data)
  Fz FL/1(TV_Info) -> Mux/1  "Fz_FL"
  Fz FR/1(TV_Info) -> Mux/2  "Fz_FR"
  Fz RL/1(TV_Info) -> Mux/3  "Fz_RL"
  Fz RR/1(TV_Info) -> Mux/4  "Fz_RR"
  Mux/1 -> Fz [4x1]/1

== system TVModel/Subsystem/Subsystem1/Slip Control/Traction Control/Subsystem/Load Transfer Calculation1 ==
  In Bus Element : Inport  PortName=dynamics_data
  Fz FL : Subsystem
  Fz FR : Subsystem
  Fz RL : Subsystem
  Fz RR : Subsystem
  Mux : Mux
  Fz [4x1] : Outport
  wires:
  Mux/1 -> Fz [4x1]/1
  Fz RR/1(TV_Info) -> Mux/4  "Fz_RR"
  Fz RL/1(TV_Info) -> Mux/3  "Fz_RL"
  Fz FR/1(TV_Info) -> Mux/2  "Fz_FR"
  Fz FL/1(TV_Info) -> Mux/1  "Fz_FL"
  In Bus Element/1 -> Fz RR/1(dynamics_data), Fz RL/1(dynamics_data), Fz FR/1(dynamics_data), Fz FL/1(dynamics_data)

== system TVModel/Subsystem/Subsystem1/Slip Control/Traction Control/Subsystem/Subsystem ==
  Inport : Inport
  Inport1 : Inport  Port=2
  Chart : Stateflow chart  TreatAsAtomicUnit=on
  Chart1 : Stateflow chart  TreatAsAtomicUnit=on
  Chart2 : Stateflow chart  TreatAsAtomicUnit=on
  Chart3 : Stateflow chart  TreatAsAtomicUnit=on
  Demux : Demux
  Demux1 : Demux
  Mux : Mux
  Out1 : Outport
  wires:
  Chart/1(TC_max) -> Mux/1  "TC_output"
  Chart1/1(TC_max) -> Mux/2  "TC_output"
  Chart2/1(TC_max) -> Mux/3  "TC_output"
  Chart3/1(TC_max) -> Mux/4  "TC_output"
  Mux/1 -> Out1/1  "TC_output"
  Inport1/1 -> Demux/1
  Inport/1 -> Demux1/1
  Demux1/1 -> Chart/1(T_ff)
  Demux1/2 -> Chart1/1(T_ff)
  Demux1/3 -> Chart2/1(T_ff)
  Demux1/4 -> Chart3/1(T_ff)
  Demux/4 -> Chart3/2(epsilon)
  Demux/3 -> Chart2/2(epsilon)
  Demux/2 -> Chart1/2(epsilon)
  Demux/1 -> Chart/2(epsilon)

== system TVModel/Subsystem/Subsystem1/Slip Control/Traction Control/Subsystem1/Load Transfer Calculation ==
  In Bus Element : Inport  PortName=dynamics_data
  Fz FL : Subsystem
  Fz FR : Subsystem
  Fz RL : Subsystem
  Fz RR : Subsystem
  Mux : Mux
  Fz [4x1] : Outport
  wires:
  In Bus Element/1 -> Fz FL/1(dynamics_data), Fz FR/1(dynamics_data), Fz RL/1(dynamics_data), Fz RR/1(dynamics_data)
  Fz FL/1(TV_Info) -> Mux/1  "Fz_FL"
  Fz FR/1(TV_Info) -> Mux/2  "Fz_FR"
  Fz RL/1(TV_Info) -> Mux/3  "Fz_RL"
  Fz RR/1(TV_Info) -> Mux/4  "Fz_RR"
  Mux/1 -> Fz [4x1]/1

== system TVModel/Subsystem/Subsystem1/Slip Control/Traction Control/Subsystem1/Load Transfer Calculation1 ==
  In Bus Element : Inport  PortName=dynamics_data
  Fz FL : Subsystem
  Fz FR : Subsystem
  Fz RL : Subsystem
  Fz RR : Subsystem
  Mux : Mux
  Fz [4x1] : Outport
  wires:
  Mux/1 -> Fz [4x1]/1
  Fz RR/1(TV_Info) -> Mux/4  "Fz_RR"
  Fz RL/1(TV_Info) -> Mux/3  "Fz_RL"
  Fz FR/1(TV_Info) -> Mux/2  "Fz_FR"
  Fz FL/1(TV_Info) -> Mux/1  "Fz_FL"
  In Bus Element/1 -> Fz RR/1(dynamics_data), Fz RL/1(dynamics_data), Fz FR/1(dynamics_data), Fz FL/1(dynamics_data)

== system TVModel/Subsystem/Subsystem1/Slip Control/Traction Control/Subsystem1/Subsystem ==
  Inport : Inport
  Inport1 : Inport  Port=2
  Chart : Stateflow chart  TreatAsAtomicUnit=on
  Chart1 : Stateflow chart  TreatAsAtomicUnit=on
  Chart2 : Stateflow chart  TreatAsAtomicUnit=on
  Chart3 : Stateflow chart  TreatAsAtomicUnit=on
  Demux : Demux
  Demux1 : Demux
  Mux : Mux
  Out1 : Outport
  wires:
  Chart/1(TC_max) -> Mux/1  "TC_output"
  Chart1/1(TC_max) -> Mux/2  "TC_output"
  Chart2/1(TC_max) -> Mux/3  "TC_output"
  Chart3/1(TC_max) -> Mux/4  "TC_output"
  Mux/1 -> Out1/1  "TC_output"
  Inport1/1 -> Demux/1
  Inport/1 -> Demux1/1
  Demux1/1 -> Chart/1(T_ff)
  Demux1/2 -> Chart1/1(T_ff)
  Demux1/3 -> Chart2/1(T_ff)
  Demux1/4 -> Chart3/1(T_ff)
  Demux/4 -> Chart3/2(epsilon)
  Demux/3 -> Chart2/2(epsilon)
  Demux/2 -> Chart1/2(epsilon)
  Demux/1 -> Chart/2(epsilon)

== system TVModel/Subsystem/Subsystem1/Torque Distribution/MPC/ PRE LUDO/Brake & ESP ==
  ubu_in : Inport
  In Bus Element13 : Inport  Port=2  PortName=brake_signal  Element=regen
  Constant : Constant  Commented=on
  Constant1 : Constant  Commented=on  Value=0
  Product : Product  Commented=on
  Switch : Switch  Commented=on  Criteria=u2 > Threshold  Threshold=0.95  SaturateOnIntegerOverflow=off  InputSameDT=off
  ubu_out : Outport
  wires:
  Constant/1 -> Switch/3
  Constant1/1 -> Switch/1
  ubu_in/1 -> ubu_out/1
  Switch/1 -> Product/2
  Product/1 -> ?
  In Bus Element13/1 -> Switch/2

== system TVModel/Subsystem/Subsystem1/Torque Distribution/MPC/ PRE LUDO/Faul Detection ==
  note: Utilizzando Simple Torque OCP Status può andare sempre in OCP 4
  In1 : Inport
  OCP Status : Inport  Port=2
  Action Port : Inport  Port=3
  dynamics_data : Inport  Port=4
  dynamics_data1 : Inport  Port=5
  driver_inputs : Inport  Port=6
  brake_signal : Inport  Port=7
  In8 : Inport  Port=8
  If1 : If  Commented=on  IfExpression=u1 == 1
  MPC : Subsystem  Commented=on  TreatAsAtomicUnit=on
  Merge : Merge  Commented=on
  Selector : Selector  Commented=on  InputPortWidth=7  IndexOptions=Index vector (dialog)  Indices=[4:7]  OutputSizes=1
  Simple torque : Subsystem  Commented=on  TreatAsAtomicUnit=on
  Subsystem : Subsystem  Commented=on
  Terminator : Terminator  Commented=on
  Vectorino : Subsystem  Commented=on  TreatAsAtomicUnit=on
  Out1 : Outport
  wires:
  dynamics_data/1 -> Subsystem/2(dynamics_data)
  If1/1 -> MPC/Action
  In8/1 -> Merge/2
  Selector/1 -> MPC/1(In1)  "Torque"
  If1/2 -> Simple torque/Action
  MPC/1(Out1) -> Merge/1
  Vectorino/1(Output) -> Terminator/1
  Merge/1 -> Out1/1
  Subsystem/1(TV Mode Selection) -> If1/1
  OCP Status/1 -> Subsystem/1(OCP Status)
  In1/1 -> Selector/1
  dynamics_data1/1 -> Vectorino/1(dynamics_data)
  driver_inputs/1 -> Vectorino/2(driver_inputs)
  brake_signal/1 -> Vectorino/3(brake_signal)
  Action Port/1 -> Vectorino/Action

== system TVModel/Subsystem/Subsystem1/Torque Distribution/MPC/ PRE LUDO/Hydraulic brakes ==
  In1 : Inport
  Brake friction : Gain  Commented=on  Gain=0.8
  Braking Areas : Constant  Commented=on  Value=[TV.CAR.BrkArea_front;TV.CAR.BrkArea_front;TV.CAR.BrkArea_rear;TV.CAR.BrkArea_rear]
  Braking Disk Radii : Constant  Commented=on  Value=[TV.CAR.DiskDiameter_front;TV.CAR.DiskDiameter_front;TV.CAR.DiskDiameter_rear;TV.CAR.DiskDiameter_rear]/2
  Product : Product  Commented=on
  Product1 : Product  Commented=on
  Out1 : Outport
  wires:
  Braking Areas/1 -> Product/2
  In1/1 -> Product/1
  Brake friction/1 -> Product1/1
  Product/1 -> Brake friction/1
  Braking Disk Radii/1 -> Product1/2
  Product1/1 -> Out1/1

== system TVModel/Subsystem/Subsystem1/Torque Distribution/MPC/ PRE LUDO/Mz = 0 Bound logic ==
  In Bus Element13 : Inport  PortName=brake_signal  Element=regen
  YRD : Inport  Port=2
  In Bus Element1 : Inport  Port=3  PortName=driver_inputs  Element=throttle
  " " : Constant  Value=0.95
  "  " : Constant  Value=TV.LV.GENERAL.ThrottleThresh
  "             " : Constant  Value=TV.LV.GENERAL.YRDTresh
  AND : Logic  IconShape=distinctive  AllPortsSameDT=off  OutDataTypeStr=boolean
  AND1 : Logic  IconShape=distinctive  AllPortsSameDT=off  OutDataTypeStr=boolean
  AND2 : Logic  IconShape=distinctive  AllPortsSameDT=off  OutDataTypeStr=boolean
  Abs : Abs  SaturateOnIntegerOverflow=off
  Constant : Constant  Value=TV.LV.GENERAL.BrakeThresh
  Constant1 : Constant  Value=10
  Data Type Conversion : DataTypeConversion  OutDataTypeStr=double  SaturateOnIntegerOverflow=off  RndMeth=Floor
  Data Type Conversion1 : DataTypeConversion  OutDataTypeStr=double  SaturateOnIntegerOverflow=off  RndMeth=Floor
  Discrete FIR Filter : DiscreteFir  Coefficients=ones(1,TV.MPC.N/TV.MPC.T*0.2)
  Gain : Gain  Gain=2
  Less Than : RelationalOperator  Operator=<=  OutDataTypeStr=fixdt(1,16)  RndMeth=Simplest  InputSameDT=off
  Less Than1 : RelationalOperator  OutDataTypeStr=boolean  RndMeth=Simplest  InputSameDT=off
  Less Than2 : RelationalOperator  Operator=<  OutDataTypeStr=boolean  RndMeth=Simplest  InputSameDT=off
  Less Than3 : RelationalOperator  Operator=<  OutDataTypeStr=boolean  RndMeth=Simplest  InputSameDT=off
  Less Than4 : RelationalOperator  OutDataTypeStr=boolean  RndMeth=Simplest  InputSameDT=off
  Sum : Sum
  flag : Outport
  wires:
  Less Than/1 -> Discrete FIR Filter/1
  Constant1/1 -> Less Than4/2
  Less Than4/1 -> AND/1, AND1/2
  Discrete FIR Filter/1 -> Less Than4/1
  "  "/1 -> Less Than1/2
  "             "/1 -> Less Than/2
  Abs/1 -> Less Than/1
  YRD/1 -> Abs/1
  In Bus Element1/1 -> Less Than1/1
  Less Than1/1 -> AND/2
  In Bus Element13/1 -> Less Than3/2, Less Than2/1
  " "/1 -> Less Than2/2
  AND1/1 -> Data Type Conversion1/1
  Gain/1 -> Sum/1
  AND/1 -> Data Type Conversion/1
  Sum/1 -> flag/1
  Data Type Conversion/1 -> Sum/2
  Data Type Conversion1/1 -> Gain/1
  AND2/1 -> AND1/1
  Less Than2/1 -> AND2/1
  Less Than3/1 -> AND2/2
  Constant/1 -> Less Than3/1

== system TVModel/Subsystem/Subsystem1/Torque Distribution/MPC/ PRE LUDO/Power Calculation Post ==
  Motor_Torque : Inport  OutDataTypeStr=double  PortDimensions=4
  In Bus Element34 : Inport  Port=2  PortName=dynamics_data  Element=omega_wheels
  In Bus Element2 : Inport  Port=2  PortName=dynamics_data  Element=omega_wheels
  "     " : Gain  Gain=TV.LV.inv_efficiency
  "      " : Gain  Gain=1/TV.LV.inv_efficiency
  Divide : Product  Inputs=*/*
  Gain2 : Gain  Gain=TV.CAR.Tau
  Power to engines : Subsystem
  Saturation : Saturate  UpperLimit=19900*pi/30  LowerLimit=100*pi/30
  Sum of Elements : Sum  Inputs=+
  Switch3 : Switch  Criteria=u2 > Threshold  SaturateOnIntegerOverflow=off  InputSameDT=off
  Terminator : Terminator
  wires:
  Divide/1 -> Sum of Elements/1
  Saturation/1 -> Divide/1, Power to engines/1(omega_motor)
  Power to engines/1(Efficiency) -> "      "/1, "     "/1
  "      "/1 -> Switch3/3  "Braking"
  "     "/1 -> Switch3/1  "Driving"
  Motor_Torque/1 -> Power to engines/2(Torque), Divide/3
  In Bus Element34/1 -> Gain2/1
  Gain2/1 -> Saturation/1
  In Bus Element2/1 -> Switch3/2
  Switch3/1 -> Divide/2
  Sum of Elements/1 -> Terminator/1  "p_el_post"

== system TVModel/Subsystem/Subsystem1/Torque Distribution/MPC/ PRE LUDO/Power Calculation Pre ==
  Motor_Torque : Inport  OutDataTypeStr=double  PortDimensions=4
  In Bus Element34 : Inport  Port=2  PortName=dynamics_data  Element=omega_wheels
  In Bus Element2 : Inport  Port=2  PortName=dynamics_data  Element=omega_wheels
  "     " : Gain  Gain=TV.LV.inv_efficiency
  "      " : Gain  Gain=1/TV.LV.inv_efficiency
  Divide : Product  Inputs=*/*
  Gain2 : Gain  Gain=TV.CAR.Tau
  Power to engines : Subsystem
  Saturation : Saturate  UpperLimit=19900*pi/30  LowerLimit=100*pi/30
  Sum of Elements : Sum  Inputs=+
  Switch3 : Switch  Criteria=u2 > Threshold  SaturateOnIntegerOverflow=off  InputSameDT=off
  Terminator : Terminator
  wires:
  Power to engines/1(Efficiency) -> "      "/1, "     "/1
  "      "/1 -> Switch3/3  "Braking"
  "     "/1 -> Switch3/1  "Driving"
  Motor_Torque/1 -> Divide/3, Power to engines/2(Torque)
  In Bus Element34/1 -> Gain2/1
  Gain2/1 -> Saturation/1
  In Bus Element2/1 -> Switch3/2
  Sum of Elements/1 -> Terminator/1  "p_el_pre"
  Saturation/1 -> Divide/1, Power to engines/1(omega_motor)
  Switch3/1 -> Divide/2
  Divide/1 -> Sum of Elements/1

== system TVModel/Subsystem/Subsystem1/Torque Distribution/MPC/ PRE LUDO/Steer_activation ==
  front_wheel_angle : Inport
  Constant : Constant  Value=TV.SIGNALS.SETTINGS.MzLimit
  Product : Product
  Steer Activation : Subsystem
  Mz_Lim : Outport
  wires:
  Constant/1 -> Product/2
  Steer Activation/1(epsilon) -> Product/1  "epsilon"
  Product/1 -> Mz_Lim/1  "Mz_Lim"
  front_wheel_angle/1 -> Steer Activation/1(front_wheel_angle)

== system TVModel/Subsystem/Subsystem1/Torque Distribution/MPC/ Parameter Bus /Bus p ==
  In : Inport
  C Function : CFunction  OutputCode=|
      | int i,j;
      | for (i = 0; i < N; i++) {
      |  for (j = 0; j < np; j++) {
      |   out_x[i*np+j] = in_x[j];
      |  }
      | }
  Constant1 : Constant  Value=TV.MPC.N + 1  OutDataTypeStr=uint8  SampleTime=TV.MPC.T/TV.MPC.N
  Constant3 : Constant  Value=TV.MPC.np  OutDataTypeStr=uint8  SampleTime=TV.MPC.T/TV.MPC.N
  Rate Transition3 : RateTransition  OutPortSampleTime=TV.MPC.T/TV.MPC.N
  TV_Info : Outport
  wires:
  Constant1/1 -> C Function/2
  C Function/1 -> TV_Info/1
  Constant3/1 -> C Function/3
  Rate Transition3/1 -> C Function/1
  In/1 -> Rate Transition3/1

== system TVModel/Subsystem/Subsystem1/Torque Distribution/MPC/Faults Detection/MPC ==
  In1 : Inport
  Action Port : ActionPort  ActionPortLabel=if(u1 == 1)
  Out1 : Outport
  wires:
  In1/1 -> Out1/1

== system TVModel/Subsystem/Subsystem1/Torque Distribution/MPC/Faults Detection/Simple torque ==
  In Bus Element11 : Inport  PortName=driver_inputs
  In Bus Element10 : Inport  Port=2  PortName=dynamics_data
  In Bus Element13 : Inport  Port=3  PortName=brake_signal
  In Bus Element12 : Inport  Port=4  PortName=hv
  In Bus torque_map1 : Inport  Port=5  PortName=car_settings
  Action Port : ActionPort  ActionPortLabel=else
  No_TV : Subsystem
  Out1 : Outport
  wires:
  No_TV/1(Output) -> Out1/1
  In Bus Element11/1 -> No_TV/2(driver_inputs)
  In Bus Element10/1 -> No_TV/1(dynamics_data)
  In Bus Element12/1 -> No_TV/5(hv)
  In Bus Element13/1 -> No_TV/4(brake_signal)
  In Bus torque_map1/1 -> No_TV/3(car_settings)

== system TVModel/Subsystem/Subsystem1/Torque Distribution/MPC/Faults Detection/Subsystem ==
  OCP Status : Inport
  In Bus Element2 : Inport  Port=2  PortName=dynamics_data  Element=vx
  Backup Map : Subsystem  TreatAsAtomicUnit=on
  Constant : Constant  Value=2
  Constant1 : Constant  Value=TV.MPC.N/TV.MPC.T*0.1-1
  Discrete FIR Filter : DiscreteFir  Coefficients=ones(1,TV.MPC.N/TV.MPC.T*0.1)
  If : If  IfExpression=u1 == 0
  Less Than1 : RelationalOperator  OutDataTypeStr=boolean  RndMeth=Simplest  InputSameDT=off
  Merge : Merge
  Selected Map : Subsystem  TreatAsAtomicUnit=on
  Switch : Switch  Criteria=u2 > Threshold  Threshold=TV.LV.GENERAL.VxTresh  SaturateOnIntegerOverflow=off  InputSameDT=off
  TV Mode Selection : Outport
  wires:
  Constant/1 -> Switch/3
  Switch/1 -> TV Mode Selection/1
  In Bus Element2/1 -> Switch/2
  Merge/1 -> Switch/1
  OCP Status/1 -> Discrete FIR Filter/1
  Discrete FIR Filter/1 -> Less Than1/1
  Constant1/1 -> Less Than1/2
  Less Than1/1 -> If/1
  If/1 -> Selected Map/Action
  Selected Map/1(Out1) -> Merge/1
  If/2 -> Backup Map/Action
  Backup Map/1(Out1) -> Merge/2
